simulink model "pcssp_PowerSupplies_harness"  (R2021b)
settings: Solver=VariableStepAuto  StartTime=0.0  StopTime=10.0  RelTol=1e-3
settings Model: DataDictionary=pcssp_PowerSupplies.sldd  Creator=ravenst1  LastModifiedBy=ravenst1

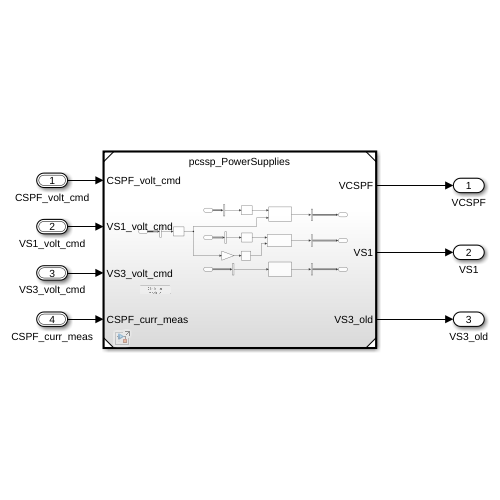
[thumbnail: Simulink's stored preview of the top-level diagram]
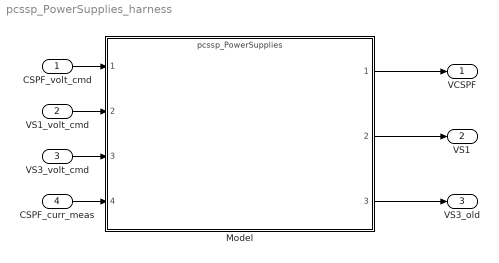
== system pcssp_PowerSupplies_harness ==
  CSPF_volt_cmd : Inport  OutDataTypeStr=Bus: pcssp_PS_CSPF_volt_cmd
  VS1_volt_cmd : Inport  Port=2  OutDataTypeStr=Bus: pcssp_PS_VS1_volt_cmd
  VS3_volt_cmd : Inport  Port=3  OutDataTypeStr=Bus: pcssp_PS_VS3_volt_cmd
  CSPF_curr_meas : Inport  Port=4  OutDataTypeStr=Bus: pcssp_PS_CSPF_curr_meas
  Model : ModelReference  ModelNameDialog=pcssp_PowerSupplies.slx  UsingDefaultArgumentValue=0  SimulationMode=Normal  ModelReferenceVersion=1.39
  VCSPF : Outport
  VS1 : Outport  Port=2
  VS3_old : Outport  Port=3
  wires:
  CSPF_volt_cmd/1 -> Model/1
  CSPF_curr_meas/1 -> Model/4
  VS3_volt_cmd/1 -> Model/3
  VS1_volt_cmd/1 -> Model/2
  Model/1 -> VCSPF/1
  Model/2 -> VS1/1
  Model/3 -> VS3_old/1
